simulink model "SOB_PMSM_Fullstate_Feedback_20241219"  (R2024b)
settings: Solver=FixedStepDiscrete  StartTime=0.0  StopTime=30  FixedStep=1/20000  RelTol=1e-3
values from neighbouring files (symbols this model uses):
  ac1_init = [a1]'    [SOB_PMSM_Fullstate_Feedback_Parameter.m]    (also in SOB_PMSM_Output_Feedback_Parameter.m)
  ac2_init = [a2]'    [SOB_PMSM_Fullstate_Feedback_Parameter.m]    (also in SOB_PMSM_Output_Feedback_Parameter.m)
  ac3_init = [a3]'    [SOB_PMSM_Fullstate_Feedback_Parameter.m]    (also in SOB_PMSM_Output_Feedback_Parameter.m)
  cr1_init = [c1]'    [SOB_PMSM_Fullstate_Feedback_Parameter.m]    (also in SOB_PMSM_Output_Feedback_Parameter.m)
  cr2_init = [c2]'    [SOB_PMSM_Fullstate_Feedback_Parameter.m]    (also in SOB_PMSM_Output_Feedback_Parameter.m)
  cr3_init = [c3]'    [SOB_PMSM_Fullstate_Feedback_Parameter.m]    (also in SOB_PMSM_Output_Feedback_Parameter.m)
  id2_init = [i2]'    [SOB_PMSM_Fullstate_Feedback_Parameter.m]    (also in SOB_PMSM_NNSMC_Parameter.m)
  id3_init = [i3]'    [SOB_PMSM_Fullstate_Feedback_Parameter.m]
  Jm = 4.675e-4    (= 0.0004675)    [SOB_PMSM_Fullstate_Feedback_Parameter.m]    (also in SOB_PMSM_NNSMC_Parameter.m; SOB_PMSM_Output_Feedback_Parameter.m)
  Km = 1.5*Psi*PolePairs    (= 0.102)    [SOB_PMSM_Fullstate_Feedback_Parameter.m]    (also in SOB_PMSM_NNSMC_Parameter.m; SOB_PMSM_Output_Feedback_Parameter.m)
undefined symbols (not defined in the file or in its folder): DiscIntNeverNeededParam
libraries: simulink x2
settings Model: Creator=COLAB  LastModifiedBy=user
settings SolverCC: AlgebraicLoopSolver=TrustRegion
settings RTWCC: GPUComputeCapability=3.5

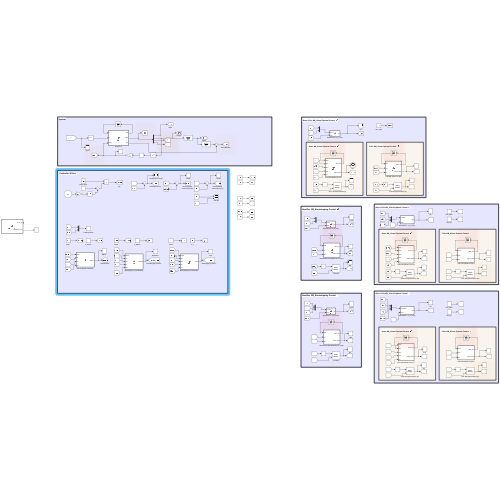
[thumbnail: Simulink's stored preview of the top-level diagram]
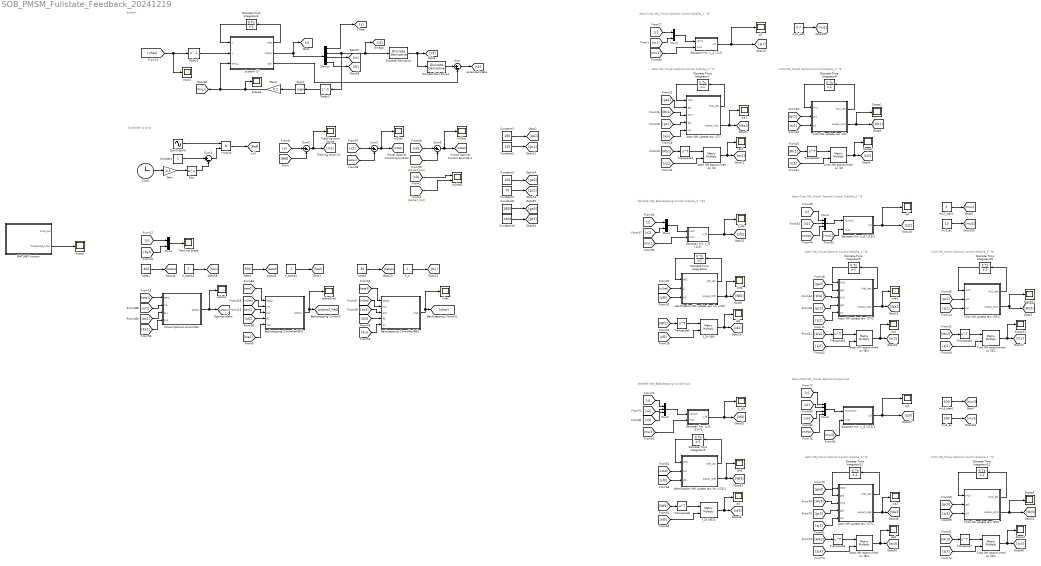
== system SOB_PMSM_Fullstate_Feedback_20241219 ==
  note: System
  note: Controller & Error
  note: Actor-Critic NN_Virtual Optimal Control $\alpha_1^*$
  note: Critic NN_Virtual Optimal Control $\alpha_1^*$
  note: Actor NN_Virtual Optimal Control $\alpha_1^*$
  note: Actor-Critic NN_Virtual Optimal Control $\alpha_2^*$
  note: Critic NN_Virtual Optimal Control $\alpha_1^*$
  note: Actor NN_Virtual Optimal Control $\alpha_1^*$
  note: Identifier NN_Backstepping Control $\alpha_2^*$$
  note: Actor-Critic NN_Virtual Optimal Control $u$
  note: Critic NN_Virtual Optimal Control $\alpha_1^*$
  note: Actor NN_Virtual Optimal Control $\alpha_1^*$
  note: Identifier NN_Backstepping Control $u$
  2sin(0.5pi*t) : Sin  Amplitude=2  Frequency=0.5*pi  SampleTime=0
  Actor NN approximation (8) : Product  Multiplication=Matrix(*)
  Actor NN approximation (8)1 : Product  Multiplication=Matrix(*)
  Actor NN approximation (8)2 : Product  Multiplication=Matrix(*)
  Actor NN update law (27) : MATLAB Function  TreatAsAtomicUnit=on
  Actor NN update law (27)1 : MATLAB Function  TreatAsAtomicUnit=on
  Actor NN update law (27)2 : MATLAB Function  TreatAsAtomicUnit=on
  Backstepping Controller(88)1 : MATLAB Function  TreatAsAtomicUnit=on
  Backstepping Controller(88)2 : MATLAB Function  TreatAsAtomicUnit=on
  Clock : Clock
  Constant : Constant
  Constant1 : Constant  Value=180
  Constant18 : Constant  Value=1400
  Constant2 : Constant  Value=140
  Constant3 : Constant  Value=100
  Constant4 : Constant  Value=70
  Constant6 : Constant  Value=1800
  Critic NN approximation (8) : Product  Multiplication=Matrix(*)
  Critic NN approximation (8)1 : Product  Multiplication=Matrix(*)
  Critic NN approximation (8)2 : Product  Multiplication=Matrix(*)
  Critic NN update law (25) : MATLAB Function  TreatAsAtomicUnit=on
  Critic NN update law (25)1 : MATLAB Function  TreatAsAtomicUnit=on
  Critic NN update law (25)2 : MATLAB Function  TreatAsAtomicUnit=on
  Delay2 : Delay  DelayLength=1
  Delay3 : Delay  DelayLength=1
  Demux : Demux
  Discrete Derivative : simulink/Discrete/Discrete Derivative  gainval=1.0  ICPrevScaledInput=0.0  OutMin=[]  OutMax=[]  OutDataType=fixdt(1, 16)  OutScaling=2^-10  DoSatur=off
  Discrete Derivative1 : simulink/Discrete/Discrete Derivative  gainval=1.0  ICPrevScaledInput=0.0  OutMin=[]  OutMax=[]  OutDataType=fixdt(1, 16)  OutScaling=2^-10  DoSatur=off
  Discrete-Time Integrator10 : DiscreteIntegrator  InitialCondition=cr2_init  SampleTime=-1  ICPrevOutput=DiscIntNeverNeededParam  ICPrevScaledInput=DiscIntNeverNeededParam
  Discrete-Time Integrator11 : DiscreteIntegrator  InitialCondition=ac3_init  SampleTime=-1  ICPrevOutput=DiscIntNeverNeededParam  ICPrevScaledInput=DiscIntNeverNeededParam
  Discrete-Time Integrator12 : DiscreteIntegrator  InitialCondition=cr3_init  SampleTime=-1  ICPrevOutput=DiscIntNeverNeededParam  ICPrevScaledInput=DiscIntNeverNeededParam
  Discrete-Time Integrator4 : DiscreteIntegrator  InitialCondition=[0 0 0 0]  SampleTime=-1  ICPrevOutput=DiscIntNeverNeededParam  ICPrevScaledInput=DiscIntNeverNeededParam
  Discrete-Time Integrator5 : DiscreteIntegrator  InitialCondition=id3_init  SampleTime=-1  ICPrevOutput=DiscIntNeverNeededParam  ICPrevScaledInput=DiscIntNeverNeededParam
  Discrete-Time Integrator6 : DiscreteIntegrator  InitialCondition=id2_init  SampleTime=-1  ICPrevOutput=DiscIntNeverNeededParam  ICPrevScaledInput=DiscIntNeverNeededParam
  Discrete-Time Integrator7 : DiscreteIntegrator  InitialCondition=ac1_init  SampleTime=-1  ICPrevOutput=DiscIntNeverNeededParam  ICPrevScaledInput=DiscIntNeverNeededParam
  Discrete-Time Integrator8 : DiscreteIntegrator  InitialCondition=cr1_init  SampleTime=-1  ICPrevOutput=DiscIntNeverNeededParam  ICPrevScaledInput=DiscIntNeverNeededParam
  Discrete-Time Integrator9 : DiscreteIntegrator  InitialCondition=ac2_init  SampleTime=-1  ICPrevOutput=DiscIntNeverNeededParam  ICPrevScaledInput=DiscIntNeverNeededParam
  Exp : Math
  Gain : Gain  Gain=-0.5
  Gain2 : Gain  Gain=0.2
  Gaussian fnc. s_f2 (114) : MATLAB Function  TreatAsAtomicUnit=on
  Gaussian fnc. s_f2 (114)1 : MATLAB Function  TreatAsAtomicUnit=on
  Gaussian fnc. s_j1 (112) : MATLAB Function  TreatAsAtomicUnit=on
  Gaussian fnc. s_j2 (115)1 : MATLAB Function  TreatAsAtomicUnit=on
  Gaussian fnc. s_j2 (115)2 : MATLAB Function  TreatAsAtomicUnit=on
  K_alpha1 : Constant
  K_alpha2 : Constant
  K_u : Constant
  MATLAB Function : MATLAB Function  TreatAsAtomicUnit=on
  Mux1 : Mux  Inputs=2
  Mux2 : Mux  Inputs=3
  Mux3 : Mux  Inputs=2
  Mux4 : Mux  Inputs=2
  Mux5 : Mux  Inputs=3
  Mux6 : Mux
  Product : Product
  S_id2 : Scope
  S_id3 : Scope
  Scope{,1..2,4,6..7,11..12} (8 alike) : Scope
  Sign2 : Signum
  Sum{,2..3,5..6} (5 alike) : Sum  Inputs=|+-
  System (1) : MATLAB Function  TreatAsAtomicUnit=on
  Tracking Scope : Scope
  Tracking error Scope : Scope
  Transpose{1..8} (8 alike) : Math  Operator=transpose  SignedPower=on
  Virtual Optimal control(26) : MATLAB Function  TreatAsAtomicUnit=on
  Wf2 : Scope
  Wf3 : Scope
  ac1 : Scope
  ac2 : Scope
  ac3 : Scope
  alpha1 : Scope
  alpha2hat : Scope
  beta1 : Constant  Value=300
  beta2 : Constant  Value=900
  beta3 : Constant  Value=30
  f_2h (86) : Product  Multiplication=Matrix(*)
  f_2h (86)1 : Product  Multiplication=Matrix(*)
  id2 : Scope
  id3 : Scope
  identification NN update law for u(23) : MATLAB Function  TreatAsAtomicUnit=on
  identification NN update law for u(23)1 : MATLAB Function  TreatAsAtomicUnit=on
  input1 : Scope
  m2hat : Scope
  m2hat2 : Scope  NumInputPorts=2
  m3hat : Scope
  mu1_iden : Constant  Value=0.7
  mu2_ac : Constant  Value=10
  mu2_iden1 : Constant  Value=2
  mu3_ac : Constant  Value=300
  mu3_iden1 : Constant  Value=400
  sj1 : Scope
  sj2 : Scope
  sj3 : Scope
  uhat : Scope
  wa1 : Scope
  wa2 : Scope
  wa3 : Scope
  wires:
  Constant1/1 -> [ga1]
  Virtual Optimal control(26)/1(alpha1) -> alpha1/1, [alpha1]
  [ac1] -> Virtual Optimal control(26)/3(ac1)
  [m1] -> Virtual Optimal control(26)/2(m1)
  [ac2] -> Backstepping Controller(88)2/3(ac2)
  [m2hat] -> Backstepping Controller(88)2/2(m2)
  beta1/1 -> [beta1]
  beta2/1 -> [beta2]
  [beta1] -> Virtual Optimal control(26)/1(beta1)
  [beta2] -> Backstepping Controller(88)2/1(beta2)
  K_alpha1/1 -> [Ka1]
  K_alpha2/1 -> [Ka2]
  [Ka1] -> Virtual Optimal control(26)/4(Ka1)
  [Ka2] -> Backstepping Controller(88)2/5(Ka2)
  Backstepping Controller(88)2/1(alpha2) -> alpha2hat/1, [alpha2_hat]
  [ga2] -> Actor NN update law (27)2/2(ga2)
  [gc2] -> Critic NN update law (25)2/2(gc2)
  Constant3/1 -> [ga2]
  Constant4/1 -> [gc2]
  [gc1] -> Critic NN update law (25)/2(gc1)
  Constant2/1 -> [gc1]
  [ga1] -> Actor NN update law (27)/2(ga1)
  Gain/1 -> Exp/1
  Sum3/1 -> Product/2
  Product/1 -> [Ref]
  Exp/1 -> Sum3/2
  Constant/1 -> Sum3/1
  Clock/1 -> Gain/1
  Gaussian fnc. s_j1 (112)/1(sj1) -> [sj1], sj1/1
  [y] -> Mux4/1
  Mux4/1 -> Gaussian fnc. s_j1 (112)/1(x1m1)
  [m1] -> Mux4/2
  [Wc1] -> Actor NN update law (27)/3(Wc1)
  [gc1] -> Actor NN update law (27)/4(gc1)
  Actor NN approximation (8)/1 -> [ac1], ac1/1
  [sj1] -> Actor NN approximation (8)/2
  Transpose3/1 -> Actor NN approximation (8)/1
  [Wa1] -> Transpose3/1
  Actor NN update law (27)/2(output_Wa1) -> wa1/1, [Wa1]
  [sj1] -> Actor NN update law (27)/5(sj1)
  Discrete-Time Integrator7/1 -> Actor NN update law (27)/1(Wa1)
  Actor NN update law (27)/1(Wa1_dot) -> Discrete-Time Integrator7/1
  Critic NN update law (25)/1(Wc1_dot) -> Discrete-Time Integrator8/1
  Discrete-Time Integrator8/1 -> Critic NN update law (25)/1(Wc1)
  [sj1] -> Critic NN update law (25)/3(sj1)
  Critic NN update law (25)/2(output_Wc1) -> [Wc1], Scope1/1
  [Wc1] -> Transpose2/1
  Transpose2/1 -> Critic NN approximation (8)/1
  [sj1] -> Critic NN approximation (8)/2
  Critic NN approximation (8)/1 -> Scope2/1, [ct1]
  [Wc2] -> Actor NN update law (27)2/3(Wc2)
  [gc2] -> Actor NN update law (27)2/4(gc2)
  Actor NN approximation (8)2/1 -> [ac2], ac2/1
  [sj2] -> Actor NN approximation (8)2/2
  Transpose1/1 -> Actor NN approximation (8)2/1
  [Wa2] -> Transpose1/1
  Actor NN update law (27)2/2(output_Wa2) -> [Wa2], wa2/1
  [sj2] -> Actor NN update law (27)2/5(sj2)
  Discrete-Time Integrator9/1 -> Actor NN update law (27)2/1(Wa2)
  Actor NN update law (27)2/1(Wa2_dot) -> Discrete-Time Integrator9/1
  Critic NN update law (25)2/1(Wc2_dot) -> Discrete-Time Integrator10/1
  Discrete-Time Integrator10/1 -> Critic NN update law (25)2/1(Wc2)
  [sj2] -> Critic NN update law (25)2/3(sj2)
  Critic NN update law (25)2/2(output_Wc2) -> Scope11/1, [Wc2]
  [Wc2] -> Transpose4/1
  Transpose4/1 -> Critic NN approximation (8)2/1
  [sj2] -> Critic NN approximation (8)2/2
  Critic NN approximation (8)2/1 -> Scope12/1, [ct2]
  [x2] -> Mux2/2
  [m2hat] -> Mux2/3
  Gaussian fnc. s_j2 (115)1/1(sj2) -> [sj2], sj2/1
  [y] -> Mux2/1
  Mux2/1 -> Gaussian fnc. s_j2 (115)1/1(x1x2m2)
  Mux3/1 -> Tracking Scope/1
  [Ref] -> Mux3/2
  [y] -> Mux3/1
  Sum2/1 -> [m1], Tracking error Scope/1
  [y] -> Sum2/1
  [Ref] -> Sum2/2
  2sin(0.5pi*t)/1 -> Product/1
  Sum5/1 -> [m2hat], m2hat/1
  [x2] -> Sum5/1
  [alpha1] -> Sum5/2
  Gaussian fnc. s_f2 (114)/1(s_f2) -> [sf2], S_id2/1
  [x2] -> Mux1/2
  Mux1/1 -> Gaussian fnc. s_f2 (114)/1(x1x2)
  [y] -> Mux1/1
  identification NN update law for u(23)/1(Wf2_dot) -> Discrete-Time Integrator6/1
  Discrete-Time Integrator6/1 -> identification NN update law for u(23)/1(Wf2)
  [m2hat] -> identification NN update law for u(23)/2(z2)
  [sf2] -> identification NN update law for u(23)/3(sf2)
  identification NN update law for u(23)/2(output_Wf2) -> [Wf2], Wf2/1
  [Wf2] -> Transpose5/1
  Transpose5/1 -> f_2h (86)/1
  [sf2] -> f_2h (86)/2
  f_2h (86)/1 -> id2/1, [id2]
  [id2] -> Backstepping Controller(88)2/4(ff2)
  [id3] -> Backstepping Controller(88)1/4(ff3)
  Backstepping Controller(88)1/1(uhat) -> [uhat], uhat/1
  [Ku] -> Backstepping Controller(88)1/5(Ku)
  K_u/1 -> [Ku]
  [beta3] -> Backstepping Controller(88)1/1(beta3)
  beta3/1 -> [beta3]
  [m3hat] -> Backstepping Controller(88)1/2(m3)
  [ac3] -> Backstepping Controller(88)1/3(ac3)
  [alpha2_hat] -> Sum6/2
  [x3] -> Sum6/1
  Sum6/1 -> m3hat/1, [m3hat]
  f_2h (86)1/1 -> [id3], id3/1
  [sf3] -> f_2h (86)1/2
  Transpose8/1 -> f_2h (86)1/1
  [Wf3] -> Transpose8/1
  identification NN update law for u(23)1/2(output_Wf3) -> Wf3/1, [Wf3]
  [sf3] -> identification NN update law for u(23)1/3(sf3)
  [m3hat] -> identification NN update law for u(23)1/2(m3)
  Discrete-Time Integrator5/1 -> identification NN update law for u(23)1/1(Wf3)
  identification NN update law for u(23)1/1(Wf3_dot) -> Discrete-Time Integrator5/1
  [y] -> Mux5/1
  Mux5/1 -> Gaussian fnc. s_f2 (114)1/1(x1x2x3)
  [x2] -> Mux5/2
  Gaussian fnc. s_f2 (114)1/1(s_f3) -> S_id3/1, [sf3]
  Mux6/1 -> Gaussian fnc. s_j2 (115)2/1(x1x2x3m3)
  [y] -> Mux6/1
  Gaussian fnc. s_j2 (115)2/1(sj3) -> sj3/1, [sj3]
  [x2] -> Mux6/2
  Critic NN approximation (8)1/1 -> [ct3], Scope7/1
  [sj3] -> Critic NN approximation (8)1/2
  Transpose7/1 -> Critic NN approximation (8)1/1
  [Wc3] -> Transpose7/1
  Critic NN update law (25)1/2(output_Wc3) -> [Wc3], Scope6/1
  [sj3] -> Critic NN update law (25)1/3(sj3)
  Discrete-Time Integrator12/1 -> Critic NN update law (25)1/1(Wc3)
  Critic NN update law (25)1/1(Wc3_dot) -> Discrete-Time Integrator12/1
  Actor NN update law (27)1/1(Wa3_dot) -> Discrete-Time Integrator11/1
  Discrete-Time Integrator11/1 -> Actor NN update law (27)1/1(Wa3)
  [sj3] -> Actor NN update law (27)1/5(sj3)
  Actor NN update law (27)1/2(output_Wa3) -> wa3/1, [Wa3]
  [Wa3] -> Transpose6/1
  Transpose6/1 -> Actor NN approximation (8)1/1
  [sj3] -> Actor NN approximation (8)1/2
  Actor NN approximation (8)1/1 -> ac3/1, [ac3]
  [gc3] -> Actor NN update law (27)1/4(gc3)
  [Wc3] -> Actor NN update law (27)1/3(Wc3)
  [gc3] -> Critic NN update law (25)1/2(gc3)
  [ga3] -> Actor NN update law (27)1/2(ga3)
  [x3] -> Mux5/3
  [m3hat] -> Mux6/4
  [x3] -> Mux6/3
  Constant18/1 -> [gc3]
  Constant6/1 -> [ga3]
  Demux/4 -> [ib]
  Demux/3 -> [ia]
  [uhat] -> Delay2/1, input1/1
  Discrete-Time Integrator4/1 -> System (1)/1(x)
  System (1)/1(xdot) -> Discrete-Time Integrator4/1
  Demux/2 -> Delay3/1, Discrete Derivative/1, [x2]
  Demux/1 -> [y]
  Sign2/1 -> Gain2/1
  Discrete Derivative/1 -> Discrete Derivative1/1, [x3]
  Gain2/1 -> System (1)/3(torq_L), [torq_L], Scope4/1
  System (1)/2(output) -> Demux/1, [x]
  Discrete Derivative1/1 -> Sum/1
  System (1)/3(g0u) -> Sum/2
  Sum/1 -> [x4]
  mu1_iden/1 -> [mu1]
  [mu1] -> Gaussian fnc. s_j1 (112)/2(mu1)
  mu2_ac/1 -> [mu2]
  [mui2] -> Gaussian fnc. s_f2 (114)/2(mu2)
  [mu2] -> Gaussian fnc. s_j2 (115)1/2(mu2)
  mu3_ac/1 -> [mu3]
  [mui3] -> Gaussian fnc. s_f2 (114)1/2(mu3)
  [mu3] -> Gaussian fnc. s_j2 (115)2/2(mu3)
  Delay2/1 -> System (1)/2(u)
  Delay3/1 -> Sign2/1
  mu2_iden1/1 -> [mui2]
  mu3_iden1/1 -> [mui3]
  [x3] -> m2hat2/1
  [alpha2_hat] -> m2hat2/2
  MATLAB Function/2(Turnaround_time) -> Scope/1

== matlab function SOB_PMSM_Fullstate_Feedback_20241219/Gaussian fnc. s_j1 (112) ==
  data: x1m1 input size=2; sj1 output size=16; mean2 parameter; mu1 input
function sj1 = fcn(x1m1,mean2, mu1)

sjm1=[0 0 0 0 0 0 0 0 0 0 0 0 0 0 0 0];

for i=1:16
    sjm1(i)=gau(i);
end

sj1 = [sjm1]';

function y = gau(x)
    y = exp(-(norm(x1m1+mean2(x,:)'))^(2)/(mu1^(2)));
end

end

== matlab function SOB_PMSM_Fullstate_Feedback_20241219/Critic NN update law (25)1 ==
  data: Wc3 input; gc3 input; sj3 input; Wc3_dot output; output_Wc3 output
function [Wc3_dot, output_Wc3] = fcn(Wc3, gc3, sj3)

Wc3_dot = -gc3*sj3*(sj3')*Wc3;

output_Wc3=Wc3;

== matlab function SOB_PMSM_Fullstate_Feedback_20241219/Gaussian fnc. s_j2 (115)1 ==
  data: x1x2m2 input size=3; sj2 output size=16; mean4 parameter; mu2 input
function sj2  = fcn(x1x2m2,mean4, mu2)

sjm2=[0 0 0 0 0 0 0 0 0 0 0 0 0 0 0 0];

for i=1:16
    sjm2(i)=gau(i);
end

sj2 = [sjm2]';

function y = gau(x)
    y = exp(-(norm(x1x2m2+mean4(x,:)'))^(2)/(mu2^(2)));
end

end

== matlab function SOB_PMSM_Fullstate_Feedback_20241219/Gaussian fnc. s_f2 (114)1 ==
  data: x1x2x3 input size=3; s_f3 output size=16; mean5 parameter; mu3 input
function s_f3 = fcn(x1x2x3,mean5, mu3)

s_fm3 = [0 0 0 0 0 0 0 0 0 0 0 0 0 0 0 0];

for i=1:16
    s_fm3(i)=gau(i);
end

s_f3 = [s_fm3]';

function y = gau(x)
    y = exp(-(norm(x1x2x3+mean5(x,:)'))^(2)/(mu3^(2)));
end

end

== matlab function SOB_PMSM_Fullstate_Feedback_20241219/identification NN update law for u(23) ==
  data: Wf2 input; z2 input; Wf2_dot output; output_Wf2 output; sf2 input
function [Wf2_dot, output_Wf2] = fcn(Wf2, z2, sf2)

GAMMA2=diag([1 1 1 1 1 1 1 1 1 1 1 1 1 1 1 1]).*(18.8);
sigma2=32.6;

Wf2_dot = [GAMMA2*(sf2*z2-sigma2*Wf2)];

output_Wf2=Wf2;

== matlab function SOB_PMSM_Fullstate_Feedback_20241219/Gaussian fnc. s_f2 (114) ==
  data: x1x2 input size=2; s_f2 output size=16; mean3 parameter; mu2 input
function s_f2 = fcn(x1x2,mean3, mu2)

s_fm2 = [0 0 0 0 0 0 0 0 0 0 0 0 0 0 0 0];

for i=1:16
    s_fm2(i)=gau(i);
end

s_f2 = [s_fm2]';

function y = gau(x)
    y = exp(-(norm(x1x2+mean3(x,:)'))^(2)/(mu2^(2)));
end

end

== matlab function SOB_PMSM_Fullstate_Feedback_20241219/Gaussian fnc. s_j2 (115)2 ==
  data: x1x2x3m3 input size=4; sj3 output size=16; mean6 parameter; mu3 input
function sj3  = fcn(x1x2x3m3,mean6, mu3)

sjm3=[0 0 0 0 0 0 0 0 0 0 0 0 0 0 0 0];

for i=1:16
    sjm3(i)=gau(i);
end

sj3 = [sjm3]';

function y = gau(x)
    y = exp(-(norm(x1x2x3m3+mean6(x,:)'))^(2)/(mu3^(2)));
end

end

== matlab function SOB_PMSM_Fullstate_Feedback_20241219/identification NN update law for u(23)1 ==
  data: Wf3 input; m3 input; Wf3_dot output; output_Wf3 output; sf3 input
function [Wf3_dot, output_Wf3] = fcn(Wf3, m3, sf3)

GAMMA2=diag([1 1 1 1 1 1 1 1 1 1 1 1 1 1 1 1]).*(136.8);
sigma2=150.6;

Wf3_dot = [GAMMA2*(sf3*m3-sigma2*Wf3)];

output_Wf3=Wf3;

== matlab function SOB_PMSM_Fullstate_Feedback_20241219/Backstepping Controller(88)2 ==
  data: beta2 input; m2 input; alpha2 output; ac2 input; ff2 input; Ka2 input; Jm parameter; Km parameter
function alpha2 = fcn(beta2, m2, ac2, ff2, Ka2, Jm, Km)

alpha2=-(Jm/Km)*(beta2*m2+ff2+(1/(2*Ka2))*ac2);%-(1/2)*(m2);

== matlab function SOB_PMSM_Fullstate_Feedback_20241219/Virtual Optimal control(26) ==
  data: beta1 input; m1 input; alpha1 output; ac1 input; Ka1 input
function alpha1 = fcn(beta1, m1, ac1, Ka1)


alpha1=-beta1*m1-(1/(2*Ka1))*ac1;%-(1/2)*(m1);

== matlab function SOB_PMSM_Fullstate_Feedback_20241219/System (1) ==
  data: x input; u input; xdot output; torq_L input; output output; g0u output
function [xdot, output, g0u] = fcn(x, u, torq_L)

Psi       = 0.017;
PolePairs = 4.0;

Km=1.5*Psi*PolePairs;
L=0.4e-3;
J=4.675e-4;
R=0.2;
P=4;
B=2.1e-3;
g0=1;

va=-u*sin(P*x(1));
vb=u*cos(P*x(1));
Omega_dot=(1/J)*(-Km*x(3)*sin(P*x(1))+Km*x(4)*cos(P*x(1))-B*x(2)-torq_L);
ia_dot=(1/L)*(va-R*x(3)+Km*x(2)*sin(P*x(1)));
ib_dot=(1/L)*(vb-R*x(4)-Km*x(2)*cos(P*x(1)));

xdot=[x(2) Omega_dot ia_dot ib_dot];

g0u=(g0*Km/(J*L))*u;
output=x;

== matlab function SOB_PMSM_Fullstate_Feedback_20241219/MATLAB Function ==
  data: time_iter output; Turnaround_time output
function [time_iter, Turnaround_time] = toggle_flag()
% time_iter: 0 또는 1로 반복적으로 변하는 출력 변수
% Turnaround_time: 측정된 작업 시간

% Persistent 변수 선언
persistent counter;
persistent stored_Turnaround_time;

% Persistent 변수 초기화
if isempty(counter)
    counter = 0; % 초기 상태 설정
end

if isempty(stored_Turnaround_time)
    stored_Turnaround_time = 0; % 초기 상태 설정
end

% 현재 상태 반환
time_iter = mod(counter, 2); % 0 또는 1을 반환

% Task Turnaround Time 측정
if time_iter == 0
    tic;
    Turnaround_time = stored_Turnaround_time; % 이전 측정값 반환
else
    stored_Turnaround_time = toc;
    Turnaround_time = stored_Turnaround_time; % 현재 측정값 반환
    fprintf('Fullstate Feedback Case Turn around time : %.12f\n', Turnaround_time);
end

% counter 증가
counter = counter + 1;

end

== matlab function SOB_PMSM_Fullstate_Feedback_20241219/Backstepping Controller(88)1 ==
  data: beta3 input; m3 input; uhat output; ac3 input; ff3 input; Ku input; L parameter
function uhat = fcn(beta3, m3, ac3, ff3, Ku, L)

uhat=-L*(beta3*m3+ff3+(1/(2*Ku))*ac3);

== matlab function SOB_PMSM_Fullstate_Feedback_20241219/Actor NN update law (27)2 ==
  data: Wa2 input; ga2 input; Wc2 input; gc2 input; sj2 input; Wa2_dot output; output_Wa2 output
function [Wa2_dot, output_Wa2] = fcn(Wa2, ga2, Wc2, gc2, sj2)

Wa2_dot = -sj2*(sj2')*((ga2*(Wa2-Wc2))+gc2*Wc2);

output_Wa2=Wa2;

== matlab function SOB_PMSM_Fullstate_Feedback_20241219/Critic NN update law (25) ==
  data: Wc1 input; gc1 input; sj1 input; Wc1_dot output; output_Wc1 output
function [Wc1_dot, output_Wc1] = fcn(Wc1, gc1, sj1)

Wc1_dot = -gc1*sj1*(sj1')*Wc1;

output_Wc1=Wc1;

== matlab function SOB_PMSM_Fullstate_Feedback_20241219/Actor NN update law (27) ==
  data: Wa1 input; ga1 input; Wc1 input; gc1 input; sj1 input; Wa1_dot output; output_Wa1 output
function [Wa1_dot, output_Wa1] = fcn(Wa1,ga1, Wc1, gc1, sj1)

Wa1_dot = -sj1*(sj1')*((ga1*(Wa1-Wc1))+gc1*Wc1);

output_Wa1=Wa1;

== matlab function SOB_PMSM_Fullstate_Feedback_20241219/Critic NN update law (25)2 ==
  data: Wc2 input; gc2 input; sj2 input; Wc2_dot output; output_Wc2 output
function [Wc2_dot, output_Wc2] = fcn(Wc2, gc2, sj2)

Wc2_dot = -gc2*sj2*(sj2')*Wc2;

output_Wc2=Wc2;

== matlab function SOB_PMSM_Fullstate_Feedback_20241219/Actor NN update law (27)1 ==
  data: Wa3 input; ga3 input; Wc3 input; gc3 input; sj3 input; Wa3_dot output; output_Wa3 output
function [Wa3_dot, output_Wa3] = fcn(Wa3, ga3, Wc3, gc3, sj3)

Wa3_dot = -sj3*(sj3')*((ga3*(Wa3-Wc3))+gc3*Wc3);

output_Wa3=Wa3;
